simulink model "Bootstrapped_Switch_v1"  (R2021b)
settings: Solver=FixedStepAuto  StartTime=0.0  StopTime=103E-6  FixedStep=200E-9  RelTol=1e-3
libraries: fl_lib x4, nesl_utility x3, ee_lib x1
settings Model: Creator=mjg65  LastModifiedBy=mjg65

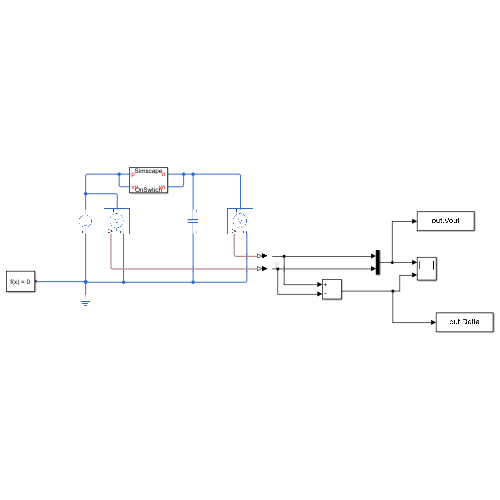
[thumbnail: Simulink's stored preview of the top-level diagram]
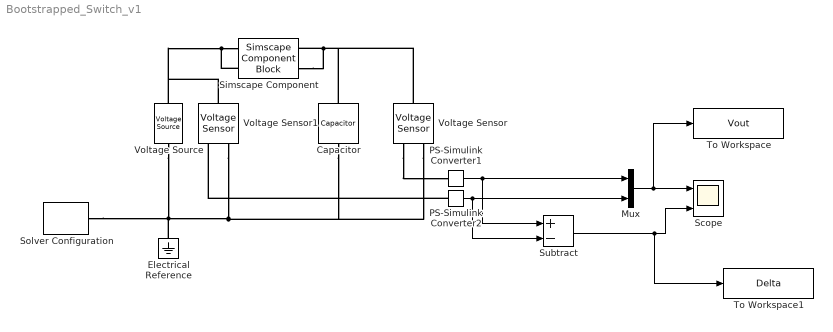
== system Bootstrapped_Switch_v1 ==
  Capacitor : fl_lib/Electrical/Electrical Elements/Capacitor  c=38.72 pF  r=0 Ohm  g=0 1/Ohm  i_specify=off  i_priority=None  i=0 A  i_nominal_specify=off  i_nominal_unit=A  i_nominal_value=1  v_specify=off  v_priority=None  v=0 V  v_nominal_specify=off  v_nominal_unit=V  v_nominal_value=1  vc_specify=off  vc_priority=High  vc=0 V  vc_nominal_specify=off  vc_nominal_unit=V  vc_nominal_value=1
  Electrical Reference : fl_lib/Electrical/Electrical Elements/Electrical Reference
  Mux : Mux  Inputs=2
  PS-Simulink Converter1 : nesl_utility/PS-Simulink Converter  PhysicalDomain=network_engine_domain  SubClassName=ps_output  LeftPortType=input  RightPortType=output  PseudoPeriodic=off  Frequencies=[]  Unit=inherit  AffineConversion=off
      settings: SourceProductBaseCode=PW,SS
  PS-Simulink Converter2 : nesl_utility/PS-Simulink Converter  PhysicalDomain=network_engine_domain  SubClassName=ps_output  LeftPortType=input  RightPortType=output  PseudoPeriodic=off  Frequencies=[]  Unit=inherit  AffineConversion=off
      settings: SourceProductBaseCode=PW,SS
  Scope : Scope  NumInputPorts=2
  Simscape Component : SimscapeComponentBlock  SourceFile=OnSwtich  ComponentPath=OnSwtich  ComponentVariants="[\"OnSwtich\"]"  ComponentVariantNames="[\"OnSwtich\"]"  ClassName=OnSwtich  SchemaVersion=1  vbs=1.8 V  vth=0.56 V  K=238.0 V^2/A  i_specify=off  i_priority=None  i=0 A  i_nominal_specify=off  i_nominal_unit=A  i_nominal_value=1  i2_specify=off  i2_priority=None  i2=0 A  i2_nominal_specify=off  i2_nominal_unit=A  i2_nominal_value=1  vsd_specify=off  vsd_priority=None  vsd=0 V  vsd_nominal_specify=off  vsd_nominal_unit=V  vsd_nominal_value=1  v_specify=off  v_priority=None  v=0 V  v_nominal_specify=off  v_nominal_unit=V  v_nominal_value=1
      settings: CopyFcn=simscape.engine.sli.internal.componentblockcallback(gcbh,'COPY')  PreCopyFcn=simscape.engine.sli.internal.componentblockcallback(gcbh,'PRECOPY')  PreDeleteFcn=simscape.engine.sli.internal.componentblockcallback(gcbh,'PREDELETE')  InternalSimscapePortConfiguration="{\"Bottom\":[],\"Left\":[{\"id\":\"p\",\"label\":\"p\",\"type\":\"foundation.electrical.electrical\"},{\"id\":\"vp\",\"label\":\"vp\",\"type\":\"foundation.electrical.electrical\"}],\"Right\":[{\"id\":\"n\",\"label\":\"n\",\"type\":\"foundation.electrical.electrical\"},{\"id\":\"vn\",\"label\":\"vn\",\"type\":\"foundation.electrical.electrical\"}],\"Top\":[]}"
      mask Type: OnSwtich
  Solver Configuration : nesl_utility/Solver Configuration  PhysicalDomain=network_engine_domain  SubClassName=solver  LeftPortType=input  RightPortType=generic  Tones=[]  Harmonics=[]  SimulateNoise=off  Profile=off  UseLocalSampling=off  EnableSwitchedLinearOptims=on  FrequencyDomain=off  UseCCode=off  RelTol=0.001  AbsTol=1e-06  MinStep=1e-09  ToWorkspace=off  RevertToSquareIcSolve=off  NumHomotopyIterations=100  PhasorMode=off  PhasorModeNumHarmonics=1  DoDC=off  ResidualTolerance=1e-09  UseLocalSolver=off  LocalSolverChoice=NE_BACKWARD_EULER_ADVANCER  LocalSolverSampleTime=0.001  DoFixedCost=off  MaxNonlinIter=3  MaxModeIter=2  ComputeImpulses=off  ImpulseIterations=2  LinearAlgebra=auto  EquationFormulation=NE_TIME_EF  DelaysMemoryBudget=1024  AutomaticFiltering=on  FilteringTimeConstant=0.001  PartitionStorageMethod=AS_NEEDED  PartitionMemoryBudget=1024  PartitionMethod=ROBUST
      settings: SourceProductBaseCode=PW,SS
  Subtract : Sum  Inputs=+-
  To Workspace : ToWorkspace  VariableName=Vout  SampleTime=-1
      settings: MaxDataPoints=512
  To Workspace1 : ToWorkspace  VariableName=Delta  SampleTime=-1
      settings: MaxDataPoints=512
  Voltage Sensor : fl_lib/Electrical/Electrical Sensors/Voltage Sensor
  Voltage Sensor1 : fl_lib/Electrical/Electrical Sensors/Voltage Sensor
  Voltage Source : ee_lib/Sources/Voltage Source  dc_voltage=0.9 V  ac_voltage=0.895 V  ac_shift=0 rad  ac_frequency=224609.375 Hz  noise_mode=0  PSD=0 V^2/Hz  repeatability=1  auto_seed=19669336  user_seed=0  sample_time=1e-3 s  i_specify=off  i_priority=None  i=0 A  i_nominal_specify=off  i_nominal_unit=A  i_nominal_value=1  v_specify=off  v_priority=None  v=0 V  v_nominal_specify=off  v_nominal_unit=V  v_nominal_value=1
  wires:
  PS-Simulink Converter2/1 -> Subtract/2, Mux/2
  PS-Simulink Converter1/1 -> Subtract/1, Mux/1
  Mux/1 -> To Workspace/1, Scope/1
  Subtract/1 -> To Workspace1/1, Scope/2
  connections:
  Simscape Component/LConn2 -- Voltage Sensor1/LConn1 -- Voltage Source/LConn1 -- Simscape Component/LConn1
  Solver Configuration/RConn1 -- Electrical Reference/LConn1 -- Voltage Sensor1/RConn2 -- Voltage Sensor/RConn2 -- Capacitor/RConn1 -- Voltage Source/RConn1
  Simscape Component/RConn2 -- Voltage Sensor/LConn1 -- Capacitor/LConn1 -- Simscape Component/RConn1
  Voltage Sensor/RConn1 -- PS-Simulink Converter1/LConn1
  PS-Simulink Converter2/LConn1 -- Voltage Sensor1/RConn1
